simulink model "PMSM_MARS_SMC"  (R2023b)
settings: Solver=ode3  StartTime=0.0  StopTime=0.4  RelTol=1e-4  EnableMultiTasking=on
InitFcn:
  | Ts = 1e-6;
  | 
  | R = 0.9585;
  | L = 5.25e-3;
  | flux = 0.1827;
libraries: powerlib_extras x1, spsDCVoltageSourceLib x1, spsGroundLib x1, spsPermanentMagnetSynchronousMachineLib x1, simulink x1, spsThreePhaseVIMeasurementLib x1, spsUniversalBridgeLib x1, spspowerguiLib x1
settings Model: Creator=Administrator  LastModifiedBy=Guoguo
settings SolverCC: AlgebraicLoopSolver=TrustRegion
settings DataIOCC: LimitDataPoints=on  SaveFormat=Array  SignalLoggingSaveFormat=ModelDataLogs  ReturnWorkspaceOutputs=off
settings OptimizationCC: ExpressionDepthLimit=2147483647  InitFltsAndDblsToZero=on  LifeSpan=inf
settings DebuggingCC: SaveWithParameterizedLinksMsg=none  UnderspecifiedInitializationDetection=Classic  MergeDetectMultiDrivingBlocksExec=none  SolverPrmCheckMsg=warning  MultiTaskCondExecSysMsg=none  FcnCallInpInsideContextMsg=warning  UnconnectedInputMsg=warning  UnconnectedOutputMsg=warning  UnconnectedLineMsg=warning  StateNameClashWarn=warning  SFUnexpectedBacktrackingDiag=warning  SFNoUnconditionalDefaultTransitionDiag=warning  SFExecutionAtInitializationDiag=none  ArithmeticOperatorsInVariantConditions=warning
settings HardwareCC: ProdBitPerPointer=32  ProdBitPerSizeT=32  ProdBitPerPtrDiffT=32  ProdLargestAtomicFloat=None  ProdIntDivRoundTo=Undefined  ProdEndianess=Unspecified  ProdWordSize=32  ProdHWDeviceType=32-bit Generic
settings ModelReferenceCC: EnableRefExpFcnMdlSchedulingChecks=on  PropagateSignalLabelsOutOfModel=off
settings SFSimCC: SimUseLocalCustomCode=off  CustomCodeUndefinedFunction=UseInterfaceOnly
settings RTWCC: RTWUseLocalCustomCode=off
settings CodeAppCC: StateflowObjectComments=on
settings GRTTargetCC: TargetFcnLib=ansi_tfl_tmw.mat  TargetLangStandard=C89/C90 (ANSI)  CombineOutputUpdateFcns=off  GRTInterface=on
settings ConfigComp: CovMetricSettings=dw  CovSaveCumulativeToWorkspaceVar=on  CovSaveSingleToWorkspaceVar=on  CovExternalEMLEnable=off  CovSFcnEnable=off
settings SimscapeCC: SimscapeNormalizeSystem=off

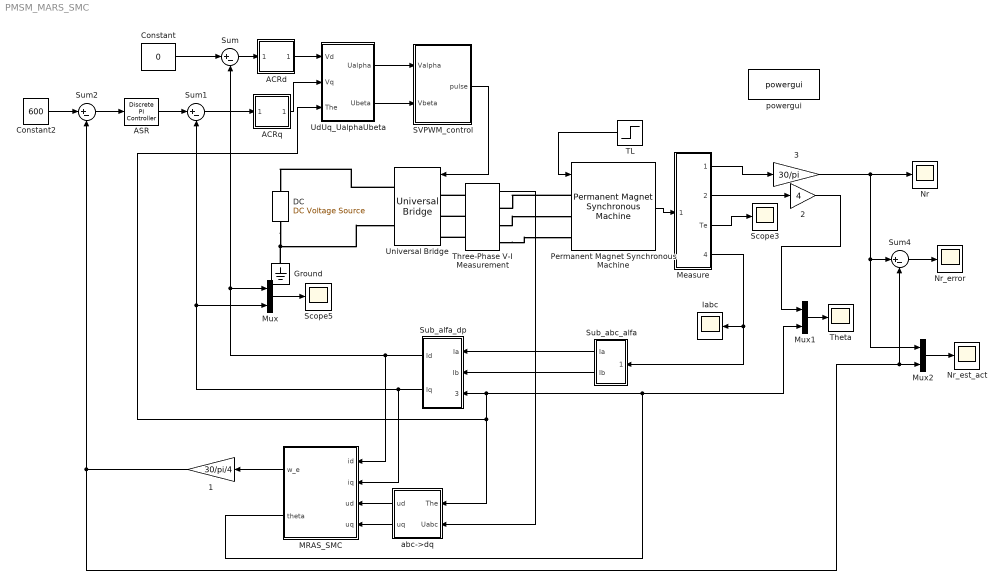
== system PMSM_MARS_SMC ==
  1 : Gain  Gain=30/pi/4
  2 : Gain  Gain=4
  3 : Gain  Gain=30/pi
  ACRd : Subsystem  mask{Kp=50, Ki=2000}
  ACRq : Subsystem  mask{Kp=50, Ki=2000}
  ASR : powerlib_extras/Discrete  Control Blocks/Discrete PI Controller  Kp=0.1  Ki=4  Par_Limits=[20 -20]  Init=0  Ts=1e-6
  Constant : Constant  Value=0
  Constant2 : Constant  Value=600
  "DC " : spsDCVoltageSourceLib/DC Voltage Source  Amplitude=300  Measurements=None
  Ground : spsGroundLib/Ground  LConnTagsString=a
  Iabc : Scope
  MRAS_SMC : Subsystem
  Measure : Subsystem
  Mux : Mux  Inputs=2
  Mux1 : Mux  Inputs=2
  Mux2 : Mux  Inputs=2
  Nr : Scope
  Nr_error : Scope
  Nr_est_act : Scope
  Permanent Magnet Synchronous Machine : spsPermanentMagnetSynchronousMachineLib/Permanent Magnet Synchronous Machine  NbPhases=3  FluxDistribution=Sinusoidal  RotorType=Salient-pole  MechanicalLoad=Torque Tm  PresetModel=No  ShowDetailedParameters=on  MeasurementBus=off  Resistance=0.9585  Inductance=8.5e-3  dqInductances=[5.25e-3,5.25e-3]  La=0.000835  MachineConstant=Flux linkage established by magnets (V.s)  Flux=0.1827  VoltageCst=132.5525  TorqueCst=1.0962  Flat=120  Mechanical=[6.329e-4 3.035e-5 4]  PolePairs=4  InitialConditions=[0,0, 0,0]  InitialConditions5ph=[0 0 0 0 0 0]  RefAngle=Aligned with phase A axis (original Park)  IterativeDiscreteModel=Trapezoidal non iterative  TsBlock=-1  TsPowergui=0
  SVPWM_control : Subsystem
  Scope3 : Scope
  Scope5 : Scope
  Sub_abc_alfa : Subsystem
  Sub_alfa_dp : Subsystem
  Sum{,1..2,4} (4 alike) : Sum  Inputs=|+-
  TL : Step  Time=.2  After=5  SampleTime=0
  Theta : Scope
  Three-Phase V-I Measurement : spsThreePhaseVIMeasurementLib/Three-Phase V-I Measurement  VoltageMeasurement=phase-to-ground  SetLabelV=off  LabelV=Vabc  Vpu=off  VpuLL=off  CurrentMeasurement=no  SetLabelI=off  LabelI=Iabc  Ipu=off  Pbase=100e6  Vbase=500e3  OutputType=Complex  PhasorSimulation=off  PSBequivalent=0
  UdUq_UalphaUbeta : Subsystem
  Universal Bridge : spsUniversalBridgeLib/Universal Bridge  Arms=3  SnubberResistance=1e5  SnubberCapacitance=inf  Device=IGBT / Diodes  Ron=1e-3  Lon=0  ForwardVoltages="[  0  0  ]"  ForwardVoltage=0  GTOparameters=[ 10e-6 , 20e-6 ]  IGBTparameters=[ 1e-6 , 2e-6 ]  Measurements=None  Measurements_2=None  converterType=Rectifier
  abc->dq : Subsystem
  powergui : spspowerguiLib/powergui  SimulationMode=Continuous  SampleTime=Ts  frequency=60  Iterations=50  frequencyindice=0  Pbase=100e6  ErrMax=1e-4  UnitsV=kV  UnitsW=MW  buscounter=0  FunctionMessages=off  echomessages=off  EnableUseOfTLC=off  CurrentSourceSwitches=on  DisableSnubberDevices=off  DisableRonSwitches=off  DisableVfSwitches=off  DisplayEquations=off  AutomaticDiscreteSolvers=off  SolverType=Tustin/Backward Euler (TBE)  Interpol=off  ExternalGateDelay=off  methode=off  Ts=0  x0status=blocks  SPID=off  SwTol=0  HookPort=off  NonlinearTolerance=1e-4  nMaxIteration=100  ContinueOnMaxIteration=off  RestoreLinks=warning  ResistiveCurrentMeasurement=off  Frange=[0:2:500]  Ylog=off  Xlog=on  ShowGrid=off  save=off  variable=ZData  structure=Iabc  ZoomFFT=on  StartTime=0.3  cycles=2  DisplayStyle=1  fundamental=40  FreqAxis=off  MaxFrequency=1000  frequencyindicesteady=1  RmsSteady=1  display=off
  wires:
  Permanent Magnet Synchronous Machine/1 -> Measure/1(In1)
  ACRd/1(Out1) -> UdUq_UalphaUbeta/1(Vd)
  Sum/1 -> ACRd/1(In1)
  Sum1/1 -> ACRq/1(In1)
  Sum2/1 -> ASR/1
  ASR/1 -> Sum1/1
  UdUq_UalphaUbeta/2(Ubeta) -> SVPWM_control/2(Vbeta)
  Measure/3(Te) -> Scope3/1
  TL/1 -> Permanent Magnet Synchronous Machine/1
  Measure/1(wm) -> 3/1
  Constant/1 -> Sum/1
  Sub_alfa_dp/1(Id) -> Sum/2, Mux/1, MRAS_SMC/1(id)
  Sub_alfa_dp/2(Iq) -> Sum1/2, Mux/2, MRAS_SMC/2(iq)
  Measure/4(Iabc) -> Iabc/1, Sub_abc_alfa/1(Iabc)
  Measure/2(The) -> 2/1
  Mux/1 -> Scope5/1
  3/1 -> Nr/1, Sum4/1, Mux2/1
  Sub_abc_alfa/1(Ia) -> Sub_alfa_dp/1(Ia)
  Sub_abc_alfa/2(Ib) -> Sub_alfa_dp/2(Ib)
  ACRq/1(Out1) -> UdUq_UalphaUbeta/2(Vq)
  Mux1/1 -> Theta/1
  MRAS_SMC/2(theta) -> Sub_alfa_dp/3(theta), UdUq_UalphaUbeta/3(The), abc->dq/1(The), Mux1/2
  Mux2/1 -> Nr_est_act/1
  Sum4/1 -> Nr_error/1
  Constant2/1 -> Sum2/1
  abc->dq/1(ud) -> MRAS_SMC/3(ud)
  abc->dq/2(uq) -> MRAS_SMC/4(uq)
  MRAS_SMC/1(w_e) -> 1/1
  1/1 -> Sum2/2, Sum4/2, Mux2/2
  2/1 -> Mux1/1
  Three-Phase V-I Measurement/1 -> abc->dq/2(Uabc)
  UdUq_UalphaUbeta/1(Ualpha) -> SVPWM_control/1(Valpha)
  SVPWM_control/1(pulse) -> Universal Bridge/1
  connections:
  "DC "/LConn1 -- Ground/LConn1 -- Universal Bridge/RConn2
  Three-Phase V-I Measurement/LConn1 -- Universal Bridge/LConn1
  Three-Phase V-I Measurement/LConn2 -- Universal Bridge/LConn2
  Three-Phase V-I Measurement/LConn3 -- Universal Bridge/LConn3
  Permanent Magnet Synchronous Machine/LConn1 -- Three-Phase V-I Measurement/RConn1
  Three-Phase V-I Measurement/RConn2 -- Permanent Magnet Synchronous Machine/LConn2
  Three-Phase V-I Measurement/RConn3 -- Permanent Magnet Synchronous Machine/LConn3
  Universal Bridge/RConn1 -- "DC "/RConn1

== system PMSM_MARS_SMC/ACRd ==
  In1 : Inport
  Add4 : Sum
  Gain : Gain  Gain=Ki
  Gain1 : Gain  Gain=Kp
  Integrator3 : Integrator
  Out1 : Outport  VectorParamsAs1DForOutWhenUnconnected=off
  wires:
  Gain1/1 -> Add4/2
  Gain/1 -> Integrator3/1
  Add4/1 -> Out1/1
  In1/1 -> Gain1/1, Gain/1
  Integrator3/1 -> Add4/1

== system PMSM_MARS_SMC/ACRq ==
  In1 : Inport
  Add4 : Sum
  Gain : Gain  Gain=Ki
  Gain1 : Gain  Gain=Kp
  Integrator3 : Integrator
  Out1 : Outport  VectorParamsAs1DForOutWhenUnconnected=off
  wires:
  Integrator3/1 -> Add4/1
  In1/1 -> Gain/1, Gain1/1
  Add4/1 -> Out1/1
  Gain/1 -> Integrator3/1
  Gain1/1 -> Add4/2

== system PMSM_MARS_SMC/MRAS_SMC ==
  id : Inport
  iq : Inport  Port=2
  ud : Inport  Port=3
  uq : Inport  Port=4
  Integrator : Integrator
  Iqd : Subsystem
  we : Subsystem
  w_e : Outport  VectorParamsAs1DForOutWhenUnconnected=off
  theta : Outport  Port=2  VectorParamsAs1DForOutWhenUnconnected=off
  wires:
  ud/1 -> Iqd/1(ud)
  uq/1 -> Iqd/2(uq)
  iq/1 -> we/2(iq)
  Iqd/1(i_d) -> we/3(i_d)
  Iqd/2(i_q) -> we/4(i_q)
  we/1(w_e) -> Integrator/1, w_e/1, Iqd/3(we)
  Integrator/1 -> theta/1
  id/1 -> we/1(id)

== system PMSM_MARS_SMC/Measure ==
  In1 : Inport
  Bus Selector : BusSelector  OutputSignals=Stator current is_a (A),Stator current is_b (A),Stator current is_c (A)
  Bus Selector1 : BusSelector  OutputSignals=Rotor speed wm (rad/s),Rotor angle thetam (rad),Electromagnetic torque Te (N*m)
  Mux : Mux  Inputs=3
  wm : Outport  VectorParamsAs1DForOutWhenUnconnected=off
  The : Outport  Port=2  VectorParamsAs1DForOutWhenUnconnected=off
  Te : Outport  Port=3  VectorParamsAs1DForOutWhenUnconnected=off
  Iabc : Outport  Port=4  VectorParamsAs1DForOutWhenUnconnected=off
  wires:
  Bus Selector/1 -> Mux/1  "<Stator current is_a (A)>"
  Bus Selector/2 -> Mux/2  "<Stator current is_b (A)>"
  Bus Selector/3 -> Mux/3  "<Stator current is_c (A)>"
  Bus Selector1/1 -> wm/1  "<Rotor speed wm (rad/s)>"
  In1/1 -> Bus Selector1/1, Bus Selector/1
  Bus Selector1/2 -> The/1  "<Rotor angle thetam (rad)>"
  Bus Selector1/3 -> Te/1  "<Electromagnetic torque Te (N*m)>"
  Mux/1 -> Iabc/1

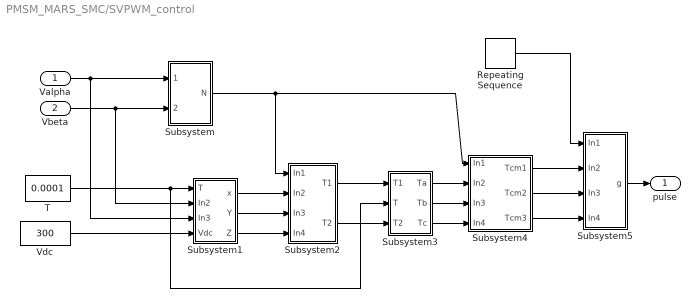
== system PMSM_MARS_SMC/SVPWM_control ==
  Valpha : Inport
  Vbeta : Inport  Port=2
  Repeating Sequence : simulink/Sources/Repeating Sequence  rep_seq_t=[0 0.00005 0.0001]  rep_seq_y=[0 0.00005 0]
  Subsystem : Subsystem
  Subsystem1 : Subsystem
  Subsystem2 : Subsystem
  Subsystem3 : Subsystem
  Subsystem4 : Subsystem
  Subsystem5 : Subsystem
  T : Constant  Value=0.0001
  Vdc : Constant  Value=300
  pulse : Outport  VectorParamsAs1DForOutWhenUnconnected=off
  wires:
  Subsystem5/1(g) -> pulse/1
  Repeating Sequence/1 -> Subsystem5/1(In1)
  Subsystem4/3(Tcm3) -> Subsystem5/4(In4)
  Subsystem4/2(Tcm2) -> Subsystem5/3(In3)
  Subsystem4/1(Tcm1) -> Subsystem5/2(In2)
  Subsystem3/3(Tc) -> Subsystem4/4(In4)
  Subsystem3/2(Tb) -> Subsystem4/3(In3)
  Subsystem3/1(Ta) -> Subsystem4/2(In2)
  Subsystem2/2(T2) -> Subsystem3/3(T2)
  Subsystem2/1(T1) -> Subsystem3/1(T1)
  Subsystem1/3(Z) -> Subsystem2/4(In4)
  Subsystem1/2(Y) -> Subsystem2/3(In3)
  Subsystem1/1(x) -> Subsystem2/2(In2)
  Subsystem/1(N) -> Subsystem4/1(In1), Subsystem2/1(In1)
  Vdc/1 -> Subsystem1/4(Vdc)
  T/1 -> Subsystem3/2(T), Subsystem1/1(T)
  Vbeta/1 -> Subsystem1/2(In2), Subsystem/2(Vbeta)
  Valpha/1 -> Subsystem1/3(In3), Subsystem/1(Valpha)

== system PMSM_MARS_SMC/Sub_abc_alfa ==
  Iabc : Inport
  Fcn : Fcn  Expr=2/3*(u(1)-0.5*u(2)-0.5*u(3))
  Fcn1 : Fcn  Expr=sqrt(1/3)*(u(2)-u(3))
  Ia : Outport  VectorParamsAs1DForOutWhenUnconnected=off
  Ib : Outport  Port=2  VectorParamsAs1DForOutWhenUnconnected=off
  wires:
  Fcn/1 -> Ia/1
  Fcn1/1 -> Ib/1
  Iabc/1 -> Fcn/1, Fcn1/1

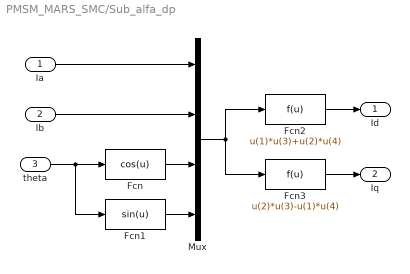
== system PMSM_MARS_SMC/Sub_alfa_dp ==
  Ia : Inport
  Ib : Inport  Port=2
  theta : Inport  Port=3
  Fcn : Fcn  Expr=cos(u)
  Fcn1 : Fcn  Expr=sin(u)
  Fcn2 : Fcn  Expr=u(1)*u(3)+u(2)*u(4)
  Fcn3 : Fcn  Expr=u(2)*u(3)-u(1)*u(4)
  Mux : Mux
  Id : Outport  VectorParamsAs1DForOutWhenUnconnected=off
  Iq : Outport  Port=2  VectorParamsAs1DForOutWhenUnconnected=off
  wires:
  theta/1 -> Fcn/1, Fcn1/1
  Ia/1 -> Mux/1
  Ib/1 -> Mux/2
  Fcn/1 -> Mux/3
  Fcn1/1 -> Mux/4
  Mux/1 -> Fcn2/1, Fcn3/1
  Fcn2/1 -> Id/1
  Fcn3/1 -> Iq/1

== system PMSM_MARS_SMC/UdUq_UalphaUbeta ==
  Vd : Inport
  Vq : Inport  Port=2
  The : Inport  Port=3
  Fcn : Fcn  Expr=cos(u[1])*u[2]-sin(u[1])*u[3]
  Fcn1 : Fcn  Expr=sin(u[1])*u[2]+cos(u[1])*u[3]
  Mux1 : Mux  Inputs=3
  Ualpha : Outport  VectorParamsAs1DForOutWhenUnconnected=off
  Ubeta : Outport  Port=2  VectorParamsAs1DForOutWhenUnconnected=off
  wires:
  Fcn1/1 -> Ubeta/1
  Fcn/1 -> Ualpha/1
  Mux1/1 -> Fcn/1, Fcn1/1
  The/1 -> Mux1/1
  Vd/1 -> Mux1/2
  Vq/1 -> Mux1/3

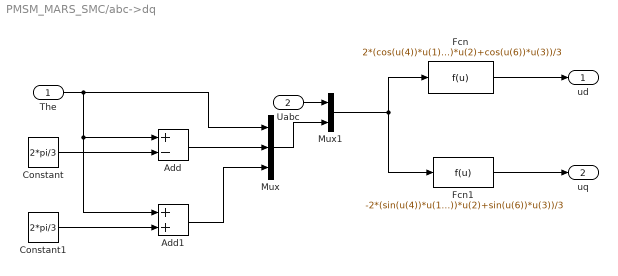
== system PMSM_MARS_SMC/abc->dq ==
  The : Inport
  Uabc : Inport  Port=2
  Add : Sum  Inputs=+-
  Add1 : Sum
  Constant : Constant  Value=2*pi/3
  Constant1 : Constant  Value=2*pi/3
  Fcn : Fcn  Expr=2*(cos(u(4))*u(1)+cos(u(5))*u(2)+cos(u(6))*u(3))/3
  Fcn1 : Fcn  Expr=-2*(sin(u(4))*u(1)+sin(u(5))*u(2)+sin(u(6))*u(3))/3
  Mux : Mux  Inputs=3
  Mux1 : Mux  Inputs=2
  ud : Outport  VectorParamsAs1DForOutWhenUnconnected=off
  uq : Outport  Port=2  VectorParamsAs1DForOutWhenUnconnected=off
  wires:
  Uabc/1 -> Mux1/1
  Fcn/1 -> ud/1
  Fcn1/1 -> uq/1
  Mux1/1 -> Fcn1/1, Fcn/1
  Mux/1 -> Mux1/2
  Add1/1 -> Mux/3
  Add/1 -> Mux/2
  The/1 -> Add/1, Add1/1, Mux/1
  Constant/1 -> Add/2
  Constant1/1 -> Add1/2

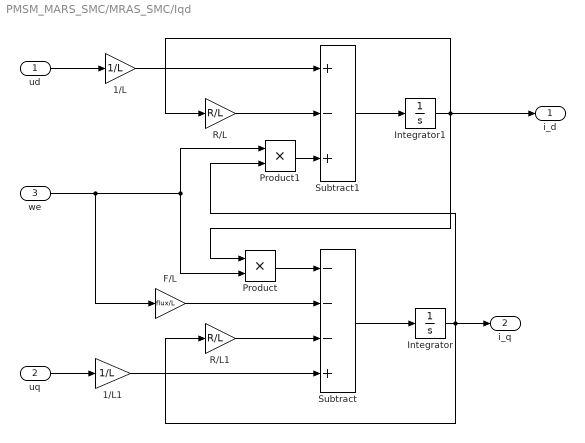
== system PMSM_MARS_SMC/MRAS_SMC/Iqd ==
  ud : Inport
  uq : Inport  Port=2
  we : Inport  Port=3
  1/L : Gain  Gain=1/L
  1/L1 : Gain  Gain=1/L
  F/L : Gain  Gain=flux/L
  Integrator : Integrator
  Integrator1 : Integrator
  Product : Product  RndMeth=Zero
  Product1 : Product  RndMeth=Zero
  R/L : Gain  Gain=R/L
  R/L1 : Gain  Gain=R/L
  Subtract : Sum  Inputs=---+
  Subtract1 : Sum  Inputs=+-+
  i_d : Outport  VectorParamsAs1DForOutWhenUnconnected=off
  i_q : Outport  Port=2  VectorParamsAs1DForOutWhenUnconnected=off
  wires:
  ud/1 -> 1/L/1
  uq/1 -> 1/L1/1
  1/L1/1 -> Subtract/4
  we/1 -> F/L/1, Product/2, Product1/1
  Subtract/1 -> Integrator/1
  Subtract1/1 -> Integrator1/1
  Integrator1/1 -> i_d/1, R/L/1, Product/1
  Integrator/1 -> i_q/1, Product1/2, R/L1/1
  1/L/1 -> Subtract1/1
  Product1/1 -> Subtract1/3
  R/L/1 -> Subtract1/2
  Product/1 -> Subtract/1
  F/L/1 -> Subtract/2
  R/L1/1 -> Subtract/3

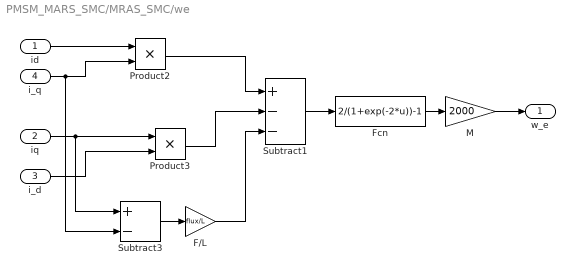
== system PMSM_MARS_SMC/MRAS_SMC/we ==
  id : Inport
  iq : Inport  Port=2
  i_d : Inport  Port=3
  i_q : Inport  Port=4
  F/L : Gain  Gain=flux/L
  Fcn : Fcn  Expr=2/(1+exp(-2*u))-1
  M : Gain  Gain=2000
  Product2 : Product  RndMeth=Zero
  Product3 : Product  RndMeth=Zero
  Subtract1 : Sum  Inputs=+--
  Subtract3 : Sum  Inputs=+-
  w_e : Outport  VectorParamsAs1DForOutWhenUnconnected=off
  wires:
  id/1 -> Product2/1
  i_q/1 -> Product2/2, Subtract3/2
  iq/1 -> Product3/1, Subtract3/1
  i_d/1 -> Product3/2
  Product2/1 -> Subtract1/1
  Product3/1 -> Subtract1/2
  Subtract3/1 -> F/L/1
  F/L/1 -> Subtract1/3
  Subtract1/1 -> Fcn/1
  Fcn/1 -> M/1
  M/1 -> w_e/1

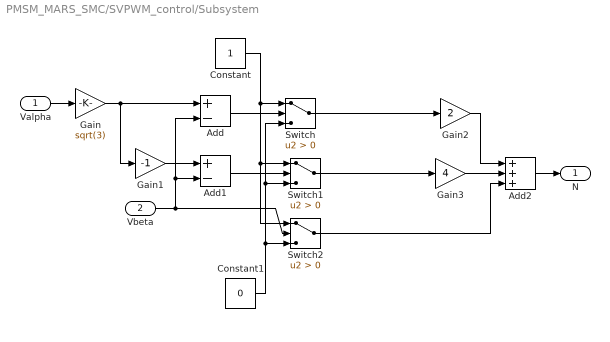
== system PMSM_MARS_SMC/SVPWM_control/Subsystem ==
  Valpha : Inport
  Vbeta : Inport  Port=2
  Add : Sum  Inputs=+-
  Add1 : Sum  Inputs=+-
  Add2 : Sum  Inputs=+++
  Constant : Constant
  Constant1 : Constant  Value=0
  Gain : Gain  Gain=sqrt(3)
  Gain1 : Gain  Gain=-1
  Gain2 : Gain  Gain=2
  Gain3 : Gain  Gain=4
  Switch : Switch  Criteria=u2 > Threshold  SaturateOnIntegerOverflow=off  InputSameDT=off
  Switch1 : Switch  Criteria=u2 > Threshold  SaturateOnIntegerOverflow=off  InputSameDT=off
  Switch2 : Switch  Criteria=u2 > Threshold  SaturateOnIntegerOverflow=off  InputSameDT=off
  N : Outport  VectorParamsAs1DForOutWhenUnconnected=off
  wires:
  Add2/1 -> N/1
  Valpha/1 -> Gain/1
  Gain3/1 -> Add2/2
  Gain2/1 -> Add2/1
  Add1/1 -> Switch1/2
  Gain1/1 -> Add1/1
  Switch1/1 -> Gain3/1
  Switch2/1 -> Add2/3
  Switch/1 -> Gain2/1
  Add/1 -> Switch/2
  Gain/1 -> Gain1/1, Add/1
  Constant1/1 -> Switch/3, Switch1/3, Switch2/3
  Constant/1 -> Switch1/1, Switch2/1, Switch/1
  Vbeta/1 -> Add1/2, Add/2, Switch2/2

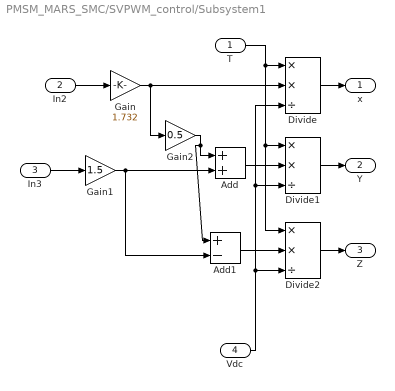
== system PMSM_MARS_SMC/SVPWM_control/Subsystem1 ==
  T : Inport
  In2 : Inport  Port=2
  In3 : Inport  Port=3
  Vdc : Inport  Port=4
  Add : Sum
  Add1 : Sum  Inputs=+-
  Divide : Product  Inputs=**/
  Divide1 : Product  Inputs=**/
  Divide2 : Product  Inputs=**/
  Gain : Gain  Gain=1.732
  Gain1 : Gain  Gain=1.5
  Gain2 : Gain  Gain=0.5
  x : Outport  VectorParamsAs1DForOutWhenUnconnected=off
  Y : Outport  Port=2  VectorParamsAs1DForOutWhenUnconnected=off
  Z : Outport  Port=3  VectorParamsAs1DForOutWhenUnconnected=off
  wires:
  Divide2/1 -> Z/1
  Divide1/1 -> Y/1
  Divide/1 -> x/1
  In3/1 -> Gain1/1
  In2/1 -> Gain/1
  Add1/1 -> Divide2/2
  Add/1 -> Divide1/2
  Gain1/1 -> Add1/2, Add/2
  Gain2/1 -> Add1/1, Add/1
  Gain/1 -> Gain2/1, Divide/2
  Vdc/1 -> Divide/3, Divide1/3, Divide2/3
  T/1 -> Divide2/1, Divide1/1, Divide/1

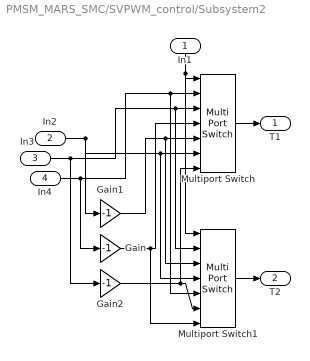
== system PMSM_MARS_SMC/SVPWM_control/Subsystem2 ==
  In1 : Inport
  In2 : Inport  Port=2
  In3 : Inport  Port=3
  In4 : Inport  Port=4
  Gain : Gain  Gain=-1
  Gain1 : Gain  Gain=-1
  Gain2 : Gain  Gain=-1
  Multiport Switch : MultiPortSwitch  Inputs=6  SaturateOnIntegerOverflow=off  InputSameDT=off
  Multiport Switch1 : MultiPortSwitch  Inputs=6  SaturateOnIntegerOverflow=off  InputSameDT=off
  T1 : Outport  VectorParamsAs1DForOutWhenUnconnected=off
  T2 : Outport  Port=2  VectorParamsAs1DForOutWhenUnconnected=off
  wires:
  Multiport Switch1/1 -> T2/1
  Multiport Switch/1 -> T1/1
  Gain2/1 -> Multiport Switch/7, Multiport Switch1/6
  Gain1/1 -> Multiport Switch1/3, Multiport Switch/5
  In2/1 -> Gain1/1, Multiport Switch/6, Multiport Switch1/4
  Gain/1 -> Multiport Switch1/7, Multiport Switch/4
  In3/1 -> Gain2/1, Multiport Switch1/2, Multiport Switch/3
  In4/1 -> Gain/1, Multiport Switch/2, Multiport Switch1/5
  In1/1 -> Multiport Switch/1, Multiport Switch1/1

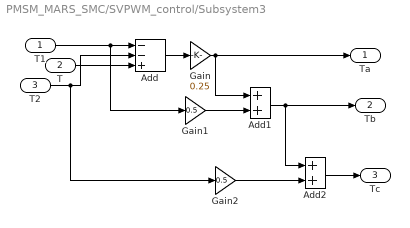
== system PMSM_MARS_SMC/SVPWM_control/Subsystem3 ==
  T1 : Inport
  T : Inport  Port=2
  T2 : Inport  Port=3
  Add : Sum  Inputs=--+
  Add1 : Sum
  Add2 : Sum
  Gain : Gain  Gain=0.25
  Gain1 : Gain  Gain=0.5
  Gain2 : Gain  Gain=0.5
  Ta : Outport  VectorParamsAs1DForOutWhenUnconnected=off
  Tb : Outport  Port=2  VectorParamsAs1DForOutWhenUnconnected=off
  Tc : Outport  Port=3  VectorParamsAs1DForOutWhenUnconnected=off
  wires:
  T/1 -> Add/3
  Add2/1 -> Tc/1
  Gain2/1 -> Add2/2
  Add1/1 -> Add2/1, Tb/1
  Gain1/1 -> Add1/2
  Gain/1 -> Add1/1, Ta/1
  Add/1 -> Gain/1
  T2/1 -> Add/2, Gain2/1
  T1/1 -> Add/1, Gain1/1

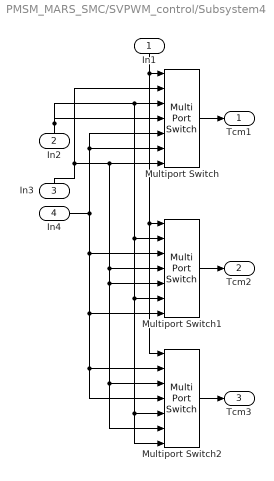
== system PMSM_MARS_SMC/SVPWM_control/Subsystem4 ==
  In1 : Inport
  In2 : Inport  Port=2
  In3 : Inport  Port=3
  In4 : Inport  Port=4
  Multiport Switch : MultiPortSwitch  Inputs=6  SaturateOnIntegerOverflow=off  InputSameDT=off
  Multiport Switch1 : MultiPortSwitch  Inputs=6  SaturateOnIntegerOverflow=off  InputSameDT=off
  Multiport Switch2 : MultiPortSwitch  Inputs=6  SaturateOnIntegerOverflow=off  InputSameDT=off
  Tcm1 : Outport  VectorParamsAs1DForOutWhenUnconnected=off
  Tcm2 : Outport  Port=2  VectorParamsAs1DForOutWhenUnconnected=off
  Tcm3 : Outport  Port=3  VectorParamsAs1DForOutWhenUnconnected=off
  wires:
  Multiport Switch2/1 -> Tcm3/1
  Multiport Switch1/1 -> Tcm2/1
  Multiport Switch/1 -> Tcm1/1
  In1/1 -> Multiport Switch2/1, Multiport Switch1/1, Multiport Switch/1
  In4/1 -> Multiport Switch1/3, Multiport Switch1/7, Multiport Switch2/2, Multiport Switch2/4, Multiport Switch/5, Multiport Switch/6
  In2/1 -> Multiport Switch/4, Multiport Switch/3, Multiport Switch1/2, Multiport Switch1/6, Multiport Switch2/5, Multiport Switch2/7
  In3/1 -> Multiport Switch/2, Multiport Switch/7, Multiport Switch1/4, Multiport Switch1/5, Multiport Switch2/3, Multiport Switch2/6

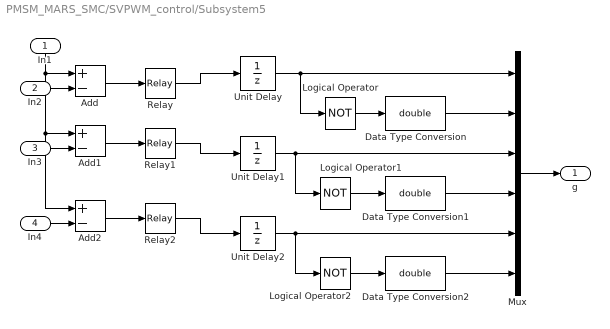
== system PMSM_MARS_SMC/SVPWM_control/Subsystem5 ==
  In1 : Inport
  In2 : Inport  Port=2
  In3 : Inport  Port=3
  In4 : Inport  Port=4
  Add : Sum  Inputs=+-
  Add1 : Sum  Inputs=+-
  Add2 : Sum  Inputs=+-
  Data Type Conversion : DataTypeConversion  OutDataTypeStr=double  SaturateOnIntegerOverflow=off  RndMeth=Floor
  Data Type Conversion1 : DataTypeConversion  OutDataTypeStr=double  SaturateOnIntegerOverflow=off  RndMeth=Floor
  Data Type Conversion2 : DataTypeConversion  OutDataTypeStr=double  SaturateOnIntegerOverflow=off  RndMeth=Floor
  Logical Operator : Logic  Operator=NOT  AllPortsSameDT=off  OutDataTypeStr=boolean
  Logical Operator1 : Logic  Operator=NOT  AllPortsSameDT=off  OutDataTypeStr=boolean
  Logical Operator2 : Logic  Operator=NOT  AllPortsSameDT=off  OutDataTypeStr=boolean
  Mux : Mux  Inputs=6
  Relay : Relay  OffSwitchValue=-eps
  Relay1 : Relay  OffSwitchValue=-eps
  Relay2 : Relay  OffSwitchValue=-eps
  Unit Delay : UnitDelay  SampleTime=-1  HasFrameUpgradeWarning=on
  Unit Delay1 : UnitDelay  SampleTime=-1  HasFrameUpgradeWarning=on
  Unit Delay2 : UnitDelay  SampleTime=-1  HasFrameUpgradeWarning=on
  g : Outport  VectorParamsAs1DForOutWhenUnconnected=off
  wires:
  In4/1 -> Add2/2
  In3/1 -> Add1/2
  In2/1 -> Add/2
  Relay2/1 -> Unit Delay2/1
  Relay1/1 -> Unit Delay1/1
  Relay/1 -> Unit Delay/1
  Unit Delay2/1 -> Mux/5, Logical Operator2/1
  Unit Delay1/1 -> Mux/3, Logical Operator1/1
  Unit Delay/1 -> Logical Operator/1, Mux/1
  Mux/1 -> g/1
  Data Type Conversion/1 -> Mux/2
  Data Type Conversion1/1 -> Mux/4
  Data Type Conversion2/1 -> Mux/6
  Logical Operator2/1 -> Data Type Conversion2/1
  Logical Operator1/1 -> Data Type Conversion1/1
  Logical Operator/1 -> Data Type Conversion/1
  Add1/1 -> Relay1/1
  Add2/1 -> Relay2/1
  Add/1 -> Relay/1
  In1/1 -> Add/1, Add2/1, Add1/1
